simulink model "sistema_pendolo_carrello"  (R2025b)
settings: Solver=ode15s  StartTime=0.0  StopTime=15  RelTol=1e-3
undefined symbols (not defined in the file): g, Kd, L, m, M, teta_zero
settings Model: Creator=USER  LastModifiedBy=francesco
settings SolverCC: AlgebraicLoopSolver=TrustRegion
settings DebuggingCC: UnconnectedInputMsg=warning  UnconnectedOutputMsg=warning  UnconnectedLineMsg=warning
settings ModelReferenceCC: EnableRefExpFcnMdlSchedulingChecks=on
settings RTWCC: GPUComputeCapability=3.5  DLArmComputeVersion=19.05

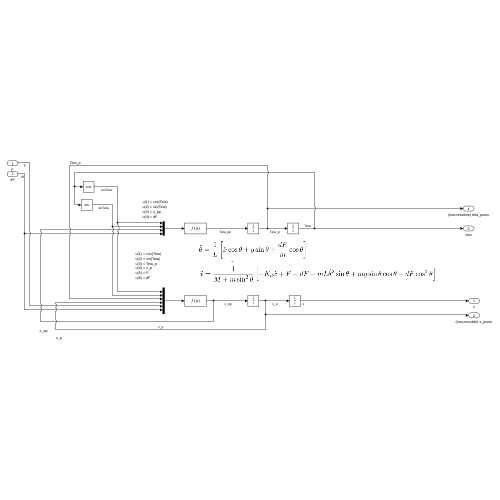
[thumbnail: Simulink's stored preview of the top-level diagram]
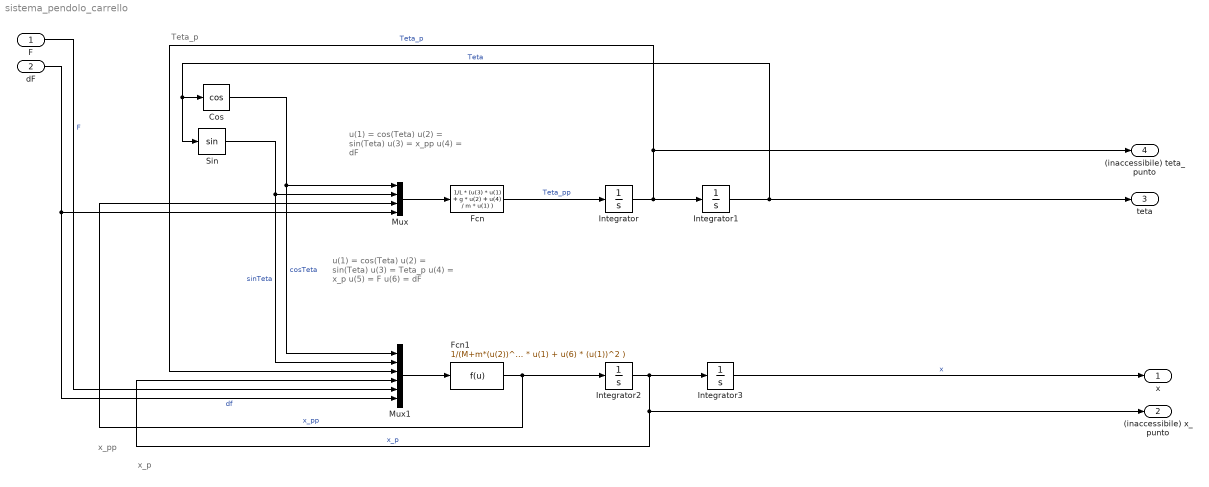
== system sistema_pendolo_carrello ==
  note: x_pp
  note: u(1) = cos(Teta)
      | u(2) = sin(Teta)
      | u(3) = x_pp
      | u(4) = dF
  note: x_p
  note: Teta_p
  note: u(1) = cos(Teta)
      | u(2) = sin(Teta)
      | u(3) = Teta_p
      | u(4) = x_p
      | u(5) = F
      | u(6) = dF
  F : Inport
  dF : Inport  Port=2
  Cos : Trigonometry  Operator=cos
  Fcn : Fcn  Expr="1/L *  (u(3) * u(1) + g * u(2) +  u(4) / m * u(1) )"
  Fcn1 : Fcn  Expr=1/(M+m*(u(2))^2 ) * ( -Kd * u(4) + u(5) - u(6) - m * L * (u(3))^2 * u(2) + m * g * u(2) * u(1) + u(6) * (u(1))^2 )
  Integrator : Integrator
  Integrator1 : Integrator  InitialCondition=teta_zero
  Integrator2 : Integrator
  Integrator3 : Integrator
  Mux : Mux
  Mux1 : Mux  Inputs=6
  Sin : Trigonometry
  x : Outport
  (inaccessibile) x_punto : Outport  Port=2
  teta : Outport  Port=3
  (inaccessibile) teta_punto : Outport  Port=4
  wires:
  Cos/1 -> Mux1/1, Mux/1  "cosTeta"
  Integrator3/1 -> x/1  "x"
  Fcn/1 -> Integrator/1  "Teta_pp"
  Integrator/1 -> Mux1/3, (inaccessibile) teta_punto/1, Integrator1/1  "Teta_p"
  F/1 -> Mux1/5  "F"
  Mux/1 -> Fcn/1
  Sin/1 -> Mux/2, Mux1/2  "sinTeta"
  Fcn1/1 -> Mux/3, Integrator2/1  "x_pp"
  Integrator1/1 -> Sin/1, Cos/1, teta/1  "Teta"
  dF/1 -> Mux/4, Mux1/6  "df"
  Integrator2/1 -> (inaccessibile) x_punto/1, Mux1/4, Integrator3/1  "x_p"
  Mux1/1 -> Fcn1/1
